simulink model "FINALPACING"  (R2020a)
settings: Solver=FixedStepAuto  StartTime=0.0  StopTime=10.0  FixedStep=1e-3  RelTol=1e-3  EnableMultiTasking=on
undefined symbols (not defined in the file): D0, D1, D10, D11, D12, D13, D2, D3, D5, D6, D8, D9, PTA0, PTA1, PTA2, PTB9, PTC16, PTC17, PTC2, PTC4, PTD0, PTD1, PTD2, PTD3
libraries: frdmk64flib x15
settings Model: ExtModeTrigDuration=5  Creator=Justin  LastModifiedBy=Justin
settings OptimizationCC: EnhancedBackFolding=on  PassReuseOutputArgsAs=Individual arguments  ZeroExternalMemoryAtStartup=off  ZeroInternalMemoryAtStartup=off  MaxStackSize=64  OptimizeBlockOrder=speed  DifferentSizesBufferReuse=on  OptimizationCustomize=off  EfficientTunableParamExpr=on
settings DebuggingCC: ParameterTunabilityLossMsg=error
settings HardwareCC: ProdBitPerPointer=32  ProdBitPerSizeT=32  ProdBitPerPtrDiffT=32  ProdLargestAtomicInteger=Long  ProdLargestAtomicFloat=Double  ProdWordSize=32  ProdHWDeviceType=ARM Compatible->ARM Cortex
settings SFSimCC: MATLABDynamicMemAlloc=off
settings RTWCC: SystemTargetFile=ert.tlc  HardwareBoard=NXP FRDM-K64F  TemplateMakefile=ert_default_tmf  Toolchain=GNU Tools for ARM Embedded Processors
settings CodeAppCC: ForceParamTrailComments=on  IgnoreCustomStorageClasses=off  OperatorAnnotations=on  SimulinkDataObjDesc=on  SFDataObjDesc=on  InsertBlockDesc=on

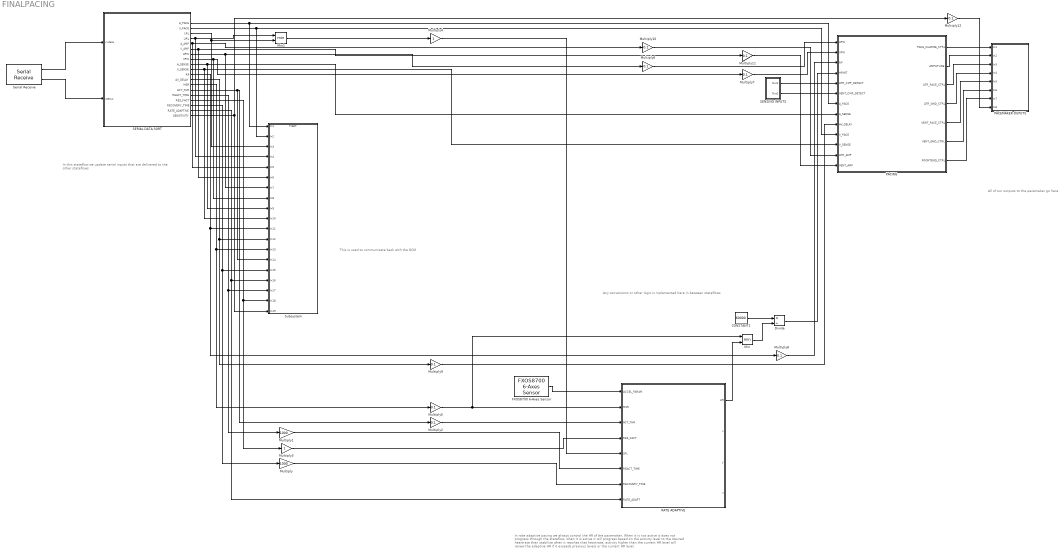
== system FINALPACING ==
  note: This is used to communicate back with the DCM
  note: In this stateflow we update serial inputs that are delivered to the
      | other stateflows
  note: In rate adaptive pacing we always control the HR of the pacemaker, When it is not active it does not progress through the stateflow, when it is active
      | it will progress based on the activity level to the desired heartrate then stabilize when it reaches that heartrate, activity higher than the current HR level
      | will renew the adaptive HR if it exceeds previous levels or the current HR level.
  note: All of our outputs to the pacemaker go here
  note: Any conversions or other logic is inplemented here in between stateflows
  CONSTANT1 : Constant  Value=60000  OutDataTypeStr=double
  Divide : Product  Inputs=*/
  FXOS8700 6-Axes Sensor : frdmk64flib/FXOS8700 6-Axes Sensor  Activesensor=Accelerometer only  ODR=800Hz  HybridODR=400Hz  Accelfullrange=-4g to +4g  SampleTime=-1
  Min : MinMax  Inputs=2
  Min1 : MinMax  Inputs=2
  Multiply : Gain  Gain=1000  ParamDataTypeStr=double
  Multiply1 : Gain  Gain=1000  ParamDataTypeStr=double
  Multiply{5..12} (8 alike) : Gain  Gain=0.1  ParamDataTypeStr=double  OutDataTypeStr=double
  Multiply2 : Gain  Gain=0.1  OutDataTypeStr=double
  Multiply3 : Gain  ParamDataTypeStr=double  OutDataTypeStr=double
  Multiply4 : Gain  ParamDataTypeStr=double  OutDataTypeStr=double
  PACEMAKER OUPUTS : Subsystem
  PACING : Stateflow chart  TreatAsAtomicUnit=on
  RATE ADAPTIVE : Stateflow chart  TreatAsAtomicUnit=on
  SENSING INPUTS : Subsystem
  SERIAL DATA SORT : Stateflow chart  TreatAsAtomicUnit=on
  Serial Receive : frdmk64flib/Serial Receive  SCIModule=0  Baudrate=uint32(9600)  Parity=None  StopBits=1  HardwareFlowControl=None  ByteOrder=LittleEndian  DataType=uint16  DataLength=24  BlockingMode=off  OutputStatus=on  SampleTime=-1
  Subsystem : Subsystem
  wires:
  Multiply11/1 -> PACING/13(VENT_AMP)
  Multiply10/1 -> PACING/12(ATR_AMP)
  SERIAL DATA SORT/17(RECOVERY_TIME) -> Multiply/1, Subsystem/15(In15)
  Min/1 -> Divide/2
  Multiply8/1 -> PACING/3(RP)
  Multiply4/1 -> RATE ADAPTIVE/5(LRL)
  SERIAL DATA SORT/12(AV_DELAY) -> Multiply9/1, Subsystem/12(In12)
  Multiply9/1 -> PACING/9(AV_DELAY)
  Multiply7/1 -> PACING/2(VPW)
  Multiply6/1 -> PACING/1(APW)
  SERIAL DATA SORT/13(MSR) -> Multiply5/1, Subsystem/13(In13)
  SERIAL DATA SORT/10(V_SENSE) -> Subsystem/10(In10), PACING/11(V_SENSE)
  Multiply2/1 -> RATE ADAPTIVE/3(ACT_THR)
  Multiply3/1 -> RATE ADAPTIVE/4(RES_FACT)
  Multiply5/1 -> Min/1, RATE ADAPTIVE/2(MSR)
  SERIAL DATA SORT/6(V_AMP) -> Multiply11/1, Subsystem/6(In6)
  Multiply/1 -> RATE ADAPTIVE/7(RECOVERY_TIME)
  SERIAL DATA SORT/3(LRL) -> Min1/2, Subsystem/3(In3)
  SERIAL DATA SORT/8(VPW) -> Multiply7/1, Subsystem/8(In8)
  FXOS8700 6-Axes Sensor/1 -> RATE ADAPTIVE/1(ACCEL_PARAM)
  SERIAL DATA SORT/5(A_AMP) -> Subsystem/5(In5), Multiply10/1
  PACING/5(VENT_PACE_CTRL) -> PACEMAKER OUPUTS/5(In5)
  PACING/2(AMPLITUDE) -> PACEMAKER OUPUTS/2(In2)
  SERIAL DATA SORT/11(RP) -> Multiply8/1, Subsystem/11(In11)
  PACING/3(ATR_PACE_CTRL) -> PACEMAKER OUPUTS/3(In3)
  PACING/7(FRONTEND_CTRL) -> PACEMAKER OUPUTS/7(In7)
  Divide/1 -> PACING/4(HRINT)
  SERIAL DATA SORT/18(RATE_ADAPTIVE) -> RATE ADAPTIVE/8(RATE_ADAPT), Subsystem/16(In16)
  PACING/1(PACE_CHARGE_CTRL) -> PACEMAKER OUPUTS/1(In1)
  SENSING INPUTS/2(Out2) -> PACING/6(VENT_CMP_DETECT)
  RATE ADAPTIVE/1(HR) -> Min/2
  SERIAL DATA SORT/19(SENSITIVITY) -> Multiply12/1, Subsystem/19(In19)
  PACING/6(VENT_GND_CTRL) -> PACEMAKER OUPUTS/6(In6)
  Min1/1 -> Multiply4/1
  SENSING INPUTS/1(Out1) -> PACING/5(ATR_CMP_DETECT)
  SERIAL DATA SORT/16(RES_FACT) -> Multiply3/1, Subsystem/18(In18)
  Serial Receive/2 -> SERIAL DATA SORT/2(status)
  PACING/4(ATR_GND_CTRL) -> PACEMAKER OUPUTS/4(In4)
  SERIAL DATA SORT/14(ACT_THR) -> Multiply2/1, Subsystem/14(In14)
  CONSTANT1/1 -> Divide/1
  Multiply1/1 -> RATE ADAPTIVE/6(REACT_TIME)
  SERIAL DATA SORT/9(A_SENSE) -> Subsystem/9(In9), PACING/8(A_SENSE)
  SERIAL DATA SORT/15(REACT_TIME) -> Multiply1/1, Subsystem/17(In17)
  SERIAL DATA SORT/4(URL) -> Min1/1, Subsystem/4(In4)
  SERIAL DATA SORT/7(APW) -> Multiply6/1, Subsystem/7(In7)
  SERIAL DATA SORT/2(V_PACE) -> PACING/10(V_PACE), Subsystem/2(In2)
  SERIAL DATA SORT/1(A_PACE) -> Subsystem/1(In1), PACING/7(A_PACE)
  Multiply12/1 -> PACEMAKER OUPUTS/8(In8)
  Serial Receive/1 -> SERIAL DATA SORT/1(rxdata)

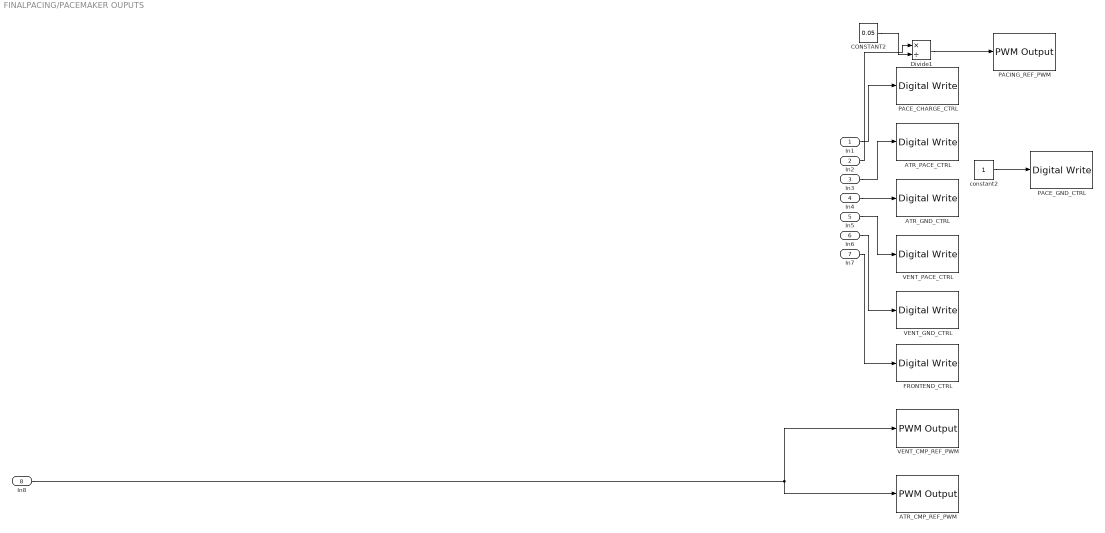
== system FINALPACING/PACEMAKER OUPUTS ==
  In1 : Inport
  In2 : Inport  Port=2
  In3 : Inport  Port=3
  In4 : Inport  Port=4
  In5 : Inport  Port=5
  In6 : Inport  Port=6
  In7 : Inport  Port=7
  In8 : Inport  Port=8
  ATR_CMP_REF_PWM : frdmk64flib/PWM Output  Whichpin=PTC2 (D6)  InitialFrequency=2000  InitialDutyCycle=0
  ATR_GND_CTRL : frdmk64flib/Digital Write  Whichpin=PTD2 (D11)
  ATR_PACE_CTRL : frdmk64flib/Digital Write  Whichpin=PTA0 (D8)
  CONSTANT2 : Constant  Value=0.05  OutDataTypeStr=double
  Divide1 : Product  Inputs=*/
  FRONTEND_CTRL : frdmk64flib/Digital Write  Whichpin=PTD1 (D13)
  PACE_CHARGE_CTRL : frdmk64flib/Digital Write  Whichpin=PTB9 (D2)
  PACE_GND_CTRL : frdmk64flib/Digital Write  Whichpin=PTD0 (D10)
  PACING_REF_PWM : frdmk64flib/PWM Output  Whichpin=PTA2 (D5)  InitialFrequency=2000  InitialDutyCycle=0
  VENT_CMP_REF_PWM : frdmk64flib/PWM Output  Whichpin=PTA1 (D3)  InitialFrequency=2000  InitialDutyCycle=0
  VENT_GND_CTRL : frdmk64flib/Digital Write  Whichpin=PTD3 (D12)
  VENT_PACE_CTRL : frdmk64flib/Digital Write  Whichpin=PTC4 (D9)
  constant2 : Constant  OutDataTypeStr=double
  wires:
  Divide1/1 -> PACING_REF_PWM/1
  In5/1 -> VENT_PACE_CTRL/1
  CONSTANT2/1 -> Divide1/2
  In8/1 -> VENT_CMP_REF_PWM/1, ATR_CMP_REF_PWM/1
  In7/1 -> FRONTEND_CTRL/1
  In2/1 -> Divide1/1
  constant2/1 -> PACE_GND_CTRL/1
  In1/1 -> PACE_CHARGE_CTRL/1
  In3/1 -> ATR_PACE_CTRL/1
  In4/1 -> ATR_GND_CTRL/1
  In6/1 -> VENT_GND_CTRL/1

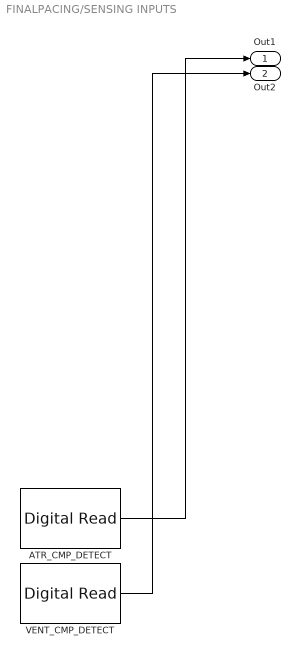
== system FINALPACING/SENSING INPUTS ==
  ATR_CMP_DETECT : frdmk64flib/Digital Read  Whichpin=PTC16 (D0)  SampleTime=-1
  VENT_CMP_DETECT : frdmk64flib/Digital Read  Whichpin=PTC17 (D1)  SampleTime=-1
  Out1 : Outport
  Out2 : Outport  Port=2
  wires:
  ATR_CMP_DETECT/1 -> Out1/1
  VENT_CMP_DETECT/1 -> Out2/1

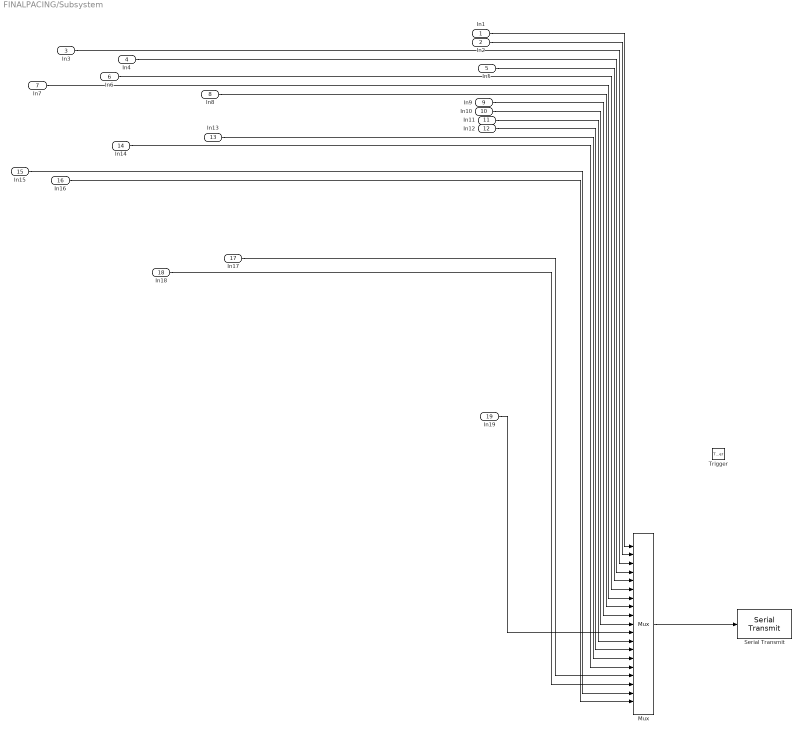
== system FINALPACING/Subsystem ==
  In1 : Inport
  In2 : Inport  Port=2
  In3 : Inport  Port=3
  In4 : Inport  Port=4
  In5 : Inport  Port=5
  In6 : Inport  Port=6
  In7 : Inport  Port=7
  In8 : Inport  Port=8
  In9 : Inport  Port=9
  In10 : Inport  Port=10
  In11 : Inport  Port=11
  In12 : Inport  Port=12
  In13 : Inport  Port=13
  In14 : Inport  Port=14
  In15 : Inport  Port=15
  In16 : Inport  Port=16
  In17 : Inport  Port=17
  In18 : Inport  Port=18
  In19 : Inport  Port=19
  Trigger : TriggerPort  TriggerType=function-call  IsSimulinkFunction=on  FunctionName=send_params  VariantControl=Variant  PortDimensions=1
  Mux : Mux  Inputs=19
  Serial Transmit : frdmk64flib/Serial Transmit  SCIModule=0  Baudrate=uint32(9600)  Parity=None  StopBits=1  HardwareFlowControl=None  ByteOrder=LittleEndian  BlockingMode=on  OutputStatus=off
  wires:
  In7/1 -> Mux/7
  In16/1 -> Mux/19
  In5/1 -> Mux/5
  Mux/1 -> Serial Transmit/1
  In1/1 -> Mux/1
  In8/1 -> Mux/8
  In2/1 -> Mux/2
  In12/1 -> Mux/13
  In18/1 -> Mux/17
  In13/1 -> Mux/14
  In6/1 -> Mux/6
  In19/1 -> Mux/11
  In4/1 -> Mux/4
  In3/1 -> Mux/3
  In11/1 -> Mux/12
  In9/1 -> Mux/9
  In10/1 -> Mux/10
  In15/1 -> Mux/18
  In17/1 -> Mux/16
  In14/1 -> Mux/15

== stateflow chart FINALPACING/RATE ADAPTIVE ==
  settings: executeAtInitialization=1
  note: Here we increment our HR by our previouslty calculated increment 100 times for the duration of the interval we calculated
      | Once we reach 100 steps we proceed into recovery time
  state ADAPTIVE_CHANGE
    entry:
    %INCREMENTING HR
    HR = HR + RATE_CHANGE_INCR
  state ADAPTIVE_RATE
    entry:
    %Calculating percentage of max activity
    PER_ACT = (x+y+z)/(MAX_ACT);
    %Calculating current percentage of activity based on HR
    PER_MAX = (HR-LRL)/(RES_FACT*MAX_CHANGE)
    %Finding Difference between the 2
    PER_ACT = PER_ACT - PER_MAX;
    %If current HR exceeds activity we return to recovery
    if PER_ACT <0
    PER_ACT =0;
    end
    %CALCULATION OF STEPS FOR INCREMENT
    RATE_CHANGE = PER_ACT*RES_FACT*MAX_CHANGE;
    RATE_CHANGE_TIME = (RATE_CHANGE/(MSR-LRL))*REACT_TIME;
    RATE_CHANGE_INCR = RATE_CHANGE/100;
    RATE_CHANGE_INTERVAL = RATE_CHANGE_TIME/100;
  state CHECK_ACTIVITY
    entry:
    %Storing accelerometer values
    x = abs(ACCEL_PARAM(1));
    y = abs(ACCEL_PARAM(2));
    z = abs(ACCEL_PARAM(3)-1);
    %RESETING DEFAULT VALUES
    HR = LRL;
    recov_count = 0;
  note: This is the initial state where we either check for activity, or maintain the LRL. This is determined by whether or not the RATE_ADAPT
      | parameter is true or false. If it is true and the activity level exceeds the threshold then we proceed into the rate adaptive HR.
  note: Here we initialize the values required to start the reactive rate adaptation. We first calculate
      | the percentage of activity we reached compared to the MAX activity we determined through
      | testing. We then find the difference between the 2 to determine how much we must adapt.
      | We then apply this percentage to the rates to determine the steps and the amount of time
      | each step should take based on our MSR and reaction time. We then proceed into the transition
  state RECOVERY_RATE
    entry:
    %CALCULATING STEPS FOR INCREMENT
    RATE_CHANGE= HR-LRL;
    RATE_CHANGE_TIME = (RATE_CHANGE/(MSR-LRL))*RECOVERY_TIME;
    RATE_CHANGE_INCR = RATE_CHANGE/100;
    RATE_CHANGE_INTERVAL = RATE_CHANGE_TIME/100;
    adapt_count = 0;
  state RECOVERY_CHANGE
    entry:
    %REDUCING HR
    HR = HR - RATE_CHANGE_INCR
  note: Here we reduce our HR while at the same time sensing if we exceed
      | our activity threshold. The values to reduce we previously calculated
      | and our sensor checks the accelerometer values. If we reach 100 steps
      | we return to our original heartrate and restart the process
  note: Here we essentaily do the same as in our adaptive rate initializaiton except with the values for recovery time.
      | Once all values are calculated we proceed into our recovey period
  RECOVERY_CHANGE -> ADAPTIVE_RATE [order 3] : [abs(ACCEL_PARAM(1))> ACT_THR || abs(ACCEL_PARAM(2))>ACT_THR || abs(ACCEL_PARAM(3)-1)> ACT_THR]{x=abs(ACCEL_PARAM(1)); y = abs(ACCEL_PARAM(2)); z = abs(ACCEL_PARAM(3)-1);}
  CHECK_ACTIVITY -> CHECK_ACTIVITY [order 2] : after(10, msec)
  (default) -> CHECK_ACTIVITY
  ADAPTIVE_RATE -> ADAPTIVE_CHANGE [order 2] : after(10, msec)
  CHECK_ACTIVITY -> ADAPTIVE_RATE [order 1] : [x > ACT_THR || y > ACT_THR ||z > ACT_THR  && RATE_ADAPT == 1]
  ADAPTIVE_CHANGE -> ADAPTIVE_CHANGE [order 1] : after(RATE_CHANGE_INTERVAL,msec){adapt_count= adapt_count+1}
  RECOVERY_CHANGE -> CHECK_ACTIVITY [order 1] : [recov_count>100]
  ADAPTIVE_CHANGE -> RECOVERY_RATE [order 2] : [adapt_count > 100]
  ADAPTIVE_RATE -> RECOVERY_RATE [order 1] : [PER_ACT == 0]
  RECOVERY_CHANGE -> RECOVERY_CHANGE [order 2] : after(RATE_CHANGE_INTERVAL,msec){recov_count = recov_count+1}
  RECOVERY_RATE -> RECOVERY_CHANGE : [after(10,msec)]
  data: ACCEL_PARAM input; MAX_ACT local double =4; PER_ACT local double; RATE_CHANGE local double; MAX_CHANGE local double =9; RATE_CHANGE_TIME local double; MSR input double; ACT_THR input double; RES_FACT input double; LRL input double; REACT_TIME input double; RATE_CHANGE_INCR local double; RATE_CHANGE_INTERVAL local double; HR output double =60; recov_count local double =0; RECOVERY_TIME input double; x output; y output; z output; adapt_count local double =0; PER_MAX local double; RATE_ADAPT input uint16

== stateflow chart FINALPACING/PACING ==
  state ATRIAL_SENSING
    entry:
    %SENSE ATR
    FRONTEND_CTRL= true;
    exit:
    FRONTEND_CTRL =false;
  state VENTRICLE_SENSING
    entry:
    %SENSE VENT
    FRONTEND_CTRL= true;
    exit:
    FRONTEND_CTRL =false;
  state CHARGE_DISCHARGE
    entry:
    %Charge/Discharge ATR
    if A_PACE == 1
    ATR_PACE_CTRL=false;
    VENT_GND_CTRL = false;
    VENT_PACE_CTRL = false;
    ATR_GND_CTRL = true;
    AMPLITUDE = ATR_AMP;
    end
    %Charge/Discharge VENT
    if V_PACE ==1 && A_PACE == 0
    VENT_PACE_CTRL = false;
    ATR_PACE_CTRL=false;
    ATR_GND_CTRL = true;
    VENT_GND_CTRL = true;
    AMPLITUDE = VENT_AMP;
    end
    PACE_CHARGE_CTRL = true;
  state ATRIAL_PACE
    entry:
    %PACE ATR
    ATR_GND_CTRL = false;
    ATR_PACE_CTRL = true;
  state VENTRICLE_PACE
    entry:
    %PACE VENT
    VENT_GND_CTRL = false;
    VENT_PACE_CTRL = true;
  state AV_DELAY
    %Charge VENT
    VENT_PACE_CTRL = false;
    AMPLITUDE = VENT_AMP;
    PACE_CHARGE_CTRL = true;
  note: This system is with all states excluding ATRIAL and VENTRICLE sensing runs the DOO mode. To get other modes we send values such as
      | A_PACE or V_SENSE to determine whether to add or remove certain states from the flow. By doing this we can have a constantly running
      | pacemaker that can dynamically change to the specific mode. The parameters sent to the stateflow can completely change the transitions
  ATRIAL_SENSING -> ATRIAL_PACE [order 2] : after(HRINT - RP-APW,msec){PACE_CHARGE_CTRL = false;}
  CHARGE_DISCHARGE -> ATRIAL_SENSING [order 2] : [after(RP,msec) && A_SENSE == 1]
  ATRIAL_SENSING -> CHARGE_DISCHARGE [order 1] : [ATR_CMP_DETECT == true]
  VENTRICLE_SENSING -> VENTRICLE_PACE [order 2] : after(HRINT- RP-VPW,msec){PACE_CHARGE_CTRL = false;}
  CHARGE_DISCHARGE -> VENTRICLE_SENSING [order 3] : [after(RP,msec) && V_SENSE == 1]
  VENTRICLE_SENSING -> CHARGE_DISCHARGE [order 1] : [VENT_CMP_DETECT == true]
  (default) -> CHARGE_DISCHARGE
  CHARGE_DISCHARGE -> CHARGE_DISCHARGE [order 1] : [A_PACE == 0 && V_PACE == 0]
  CHARGE_DISCHARGE -> ATRIAL_PACE [order 4] : [after(HRINT-APW-VPW-AV_DELAY,msec) && A_PACE == 1]{PACE_CHARGE_CTRL = false;}
  ATRIAL_PACE -> CHARGE_DISCHARGE [order 2] : [after(APW,msec) && V_PACE == 0]
  ATRIAL_PACE -> AV_DELAY [order 1] : [after(APW,msec) && V_PACE == 1]{ATR_PACE_CTRL = false; ATR_GND_CTRL =true;}
  CHARGE_DISCHARGE -> VENTRICLE_PACE [order 5] : [after(HRINT-VPW,msec) && A_PACE == 0 && V_PACE == 1]{PACE_CHARGE_CTRL = false;}
  VENTRICLE_PACE -> CHARGE_DISCHARGE : after(VPW,msec)
  AV_DELAY -> VENTRICLE_PACE : after(AV_DELAY,msec){PACE_CHARGE_CTRL = false; ATR_GND_CTRL = false;}
  data: APW input double; VPW input double; RP input double; PACE_CHARGE_CTRL output boolean; AMPLITUDE output double; HRINT input double; ATR_CMP_DETECT input boolean; ATR_PACE_CTRL output boolean; ATR_GND_CTRL output boolean; VENT_CMP_DETECT input boolean; VENT_PACE_CTRL output boolean; VENT_GND_CTRL output boolean; FRONTEND_CTRL output boolean; A_PACE input uint16; A_SENSE input uint16; AV_DELAY input double; V_PACE input uint16; V_SENSE input uint16; ATR_AMP input double; VENT_AMP input double

== stateflow chart FINALPACING/SERIAL DATA SORT ==
  settings: executeAtInitialization=1
  state SET_PARAM
    A_PACE = rxdata(1);
    V_PACE = rxdata(2);
    LRL = rxdata(3);
    URL = rxdata(4);
    A_AMP = rxdata(5);
    V_AMP = rxdata(6);
    APW = rxdata(7);
    VPW = rxdata(8);
    A_SENSE = rxdata(9);
    V_SENSE = rxdata(10);
    SENSITIVITY = rxdata(11);
    RP =rxdata(12);
    AV_DELAY =rxdata(13);
    MSR = rxdata(14);
    ACT_THR = rxdata(15);
    REACT_TIME = rxdata(16);
    RES_FACT =rxdata(17);
    RECOVERY_TIME = rxdata(18);
    RATE_ADAPTIVE =rxdata(19);
  state INITIAL
    %INITIAL OFF STATE
    entry:
    A_PACE = 0;
    V_PACE =0;
    LRL = 0;
    URL = 0;
    A_AMP = 0;%x10
    V_AMP =0;%x10
    APW = 0;%x10
    VPW = 0;%x10
    A_SENSE = 0;
    V_SENSE = 0;
    RP = 0;%x10
    AV_DELAY = 0;%x10
    MSR = 0;%x10
    ACT_THR = 0;%x10
    REACT_TIME = 0;
    RES_FACT = 0;
    RECOVERY_TIME = 0;
    RATE_ADAPTIVE = 0;
    SENSITIVITY = 530;%x10
  state STANDBY
  state ECHO_PARAM
    entry:
    send_params();
  SET_PARAM -> STANDBY
  (default) -> INITIAL
  (junction 10) -> SET_PARAM [order 1] : [rxdata(21) == hex2dec('55')]
  (junction 9) -> STANDBY [order 2]
  INITIAL -> STANDBY
  STANDBY -> (junction 9) : [status == 0]
  (junction 9) -> (junction 10) [order 1] : [rxdata(20) == hex2dec('16')]
  (junction 10) -> ECHO_PARAM [order 2] : [rxdata(21) == hex2dec('22')]
  ECHO_PARAM -> STANDBY
  data: rxdata input uint16; status input uint8; A_PACE output uint16; V_PACE output uint16; LRL output uint16; URL output uint16; A_AMP output uint16; V_AMP output uint16; APW output uint16; VPW output uint16; A_SENSE output uint16; V_SENSE output uint16; RP output uint16; AV_DELAY output uint16; MSR output uint16; ACT_THR output uint16; REACT_TIME output uint16; RES_FACT output uint16; RECOVERY_TIME output uint16; RATE_ADAPTIVE output uint16; SENSITIVITY output uint16
